simulink subsystem "canards_servo"  (R2024b)
settings: Solver=VariableStepAuto  StartTime=0.0  StopTime=10.0  RelTol=1e-3
undefined symbols (not defined in the file or in its folder): act_anglelimit, act_backlash, act_deadtime, act_ratelimit, samplingrate
libraries: simulink x1, aerolibactuator x1
settings Model: Creator=joedo  LastModifiedBy=finnb

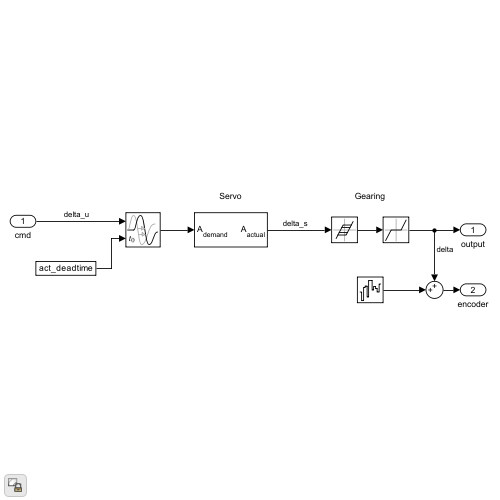
[thumbnail: Simulink's stored preview of the top-level diagram]
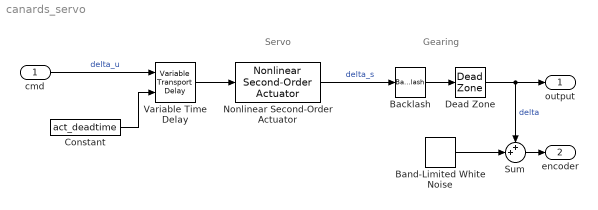
== system canards_servo ==
  note: Servo
  note: Gearing
  cmd : Inport
  Backlash : Backlash  BacklashWidth=deg2rad(act_backlash)
  Band-Limited White Noise : simulink/Sources/Band-Limited White Noise  Cov=[1e-9]  Ts=samplingrate  seed=[24563]
  Constant : Constant  Value=act_deadtime
  Dead Zone : DeadZone  LowerValue=-deg2rad(act_backlash)  UpperValue=deg2rad(act_backlash)
  Nonlinear Second-Order Actuator : aerolibactuator/Nonlinear Second-Order Actuator  wn_fin=act_freq  z_fin=act_damping  fin_max=deg2rad(act_anglelimit)  fin_min=-deg2rad(act_anglelimit)  fin_maxrate=deg2rad(act_ratelimit)  fin_act_0=0  fin_act_vel=0
  Sum : Sum  Inputs=++|
  Variable Time Delay : VariableTransportDelay  MaximumPoints=100
  output : Outport
  encoder : Outport  Port=2
  wires:
  Backlash/1 -> Dead Zone/1
  Nonlinear Second-Order Actuator/1 -> Backlash/1  "delta_s"
  Dead Zone/1 -> output/1, Sum/1  "delta"
  cmd/1 -> Variable Time Delay/1  "delta_u"
  Sum/1 -> encoder/1
  Band-Limited White Noise/1 -> Sum/2
  Variable Time Delay/1 -> Nonlinear Second-Order Actuator/1
  Constant/1 -> Variable Time Delay/2
